simulink model "sampleModel1641_2_sub"  (R2023a)
settings: Solver=VariableStepAuto  StartTime=0.0  StopTime=10.0  RelTol=1e-3
libraries: hdlsllib x4, simulink x1
settings Model: Creator=user1  LastModifiedBy=user1

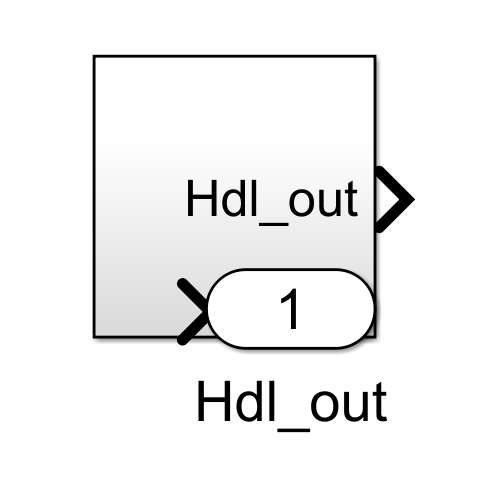
[thumbnail: Simulink's stored preview of the top-level diagram]
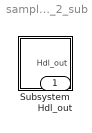
== system sampleModel1641_2_sub ==
  Subsystem : Subsystem
  Hdl_out : Outport  OutDataTypeStr=uint8

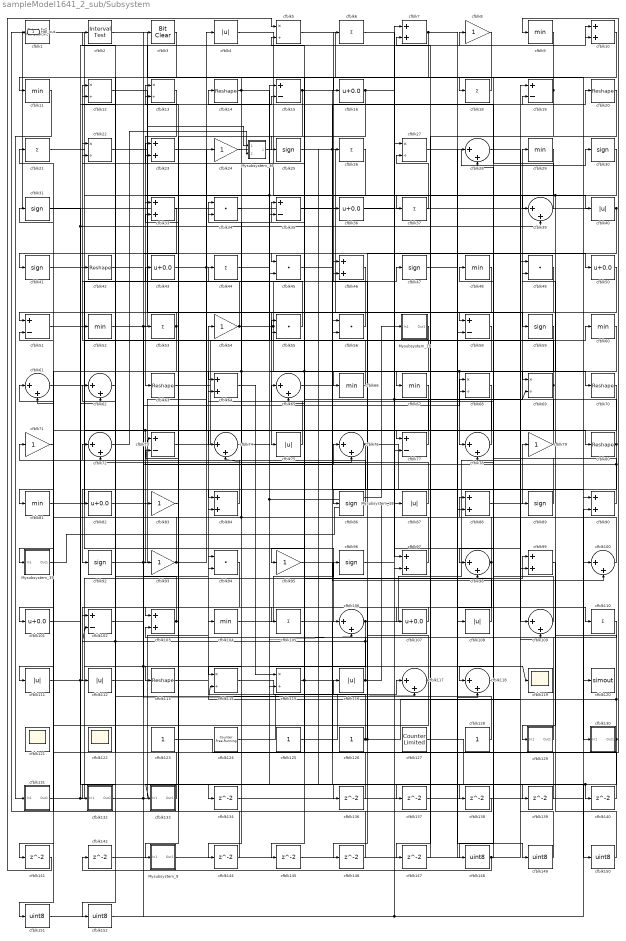
== system sampleModel1641_2_sub/Subsystem ==
  Mysubsystem_18 : Subsystem  TreatAsAtomicUnit=on  RTWFcnName=Mysubsystem_18
      settings: RTWFcnNameOpts=User specified  RTWFileNameOpts=Use function name
  Mysubsystem_19 : Subsystem  TreatAsAtomicUnit=on  RTWFcnName=Mysubsystem_19
      settings: RTWFcnNameOpts=User specified  RTWFileNameOpts=Use function name
  Mysubsystem_35 : Subsystem  TreatAsAtomicUnit=on  RTWFcnName=Mysubsystem_35
      settings: RTWFcnNameOpts=User specified  RTWFileNameOpts=Use function name
  Mysubsystem_36 : Subsystem  TreatAsAtomicUnit=on  RTWFcnName=Mysubsystem_36
      settings: RTWFcnNameOpts=User specified  RTWFileNameOpts=Use function name
  Mysubsystem_9 : Subsystem  TreatAsAtomicUnit=on  RTWFcnName=Mysubsystem_9
      settings: RTWFcnNameOpts=User specified  RTWFileNameOpts=Use function name
  cfblk1 : hdlsllib/Logic and Bit Operations/Detect Fall Nonpositive  vinit=0  OutDataTypeStr=uint8
  cfblk{7,10,23,33,46,64,84,88,90,97,99,103} (12 alike) : Sum  OutDataTypeStr=uint8
  cfblk{28,39,61..62,65,72,74,76,78,98,100,106,109,117..118} (15 alike) : Sum  Inputs=|++  OutDataTypeStr=uint8
  cfblk{16,36,43,50,82,101,107} (7 alike) : Bias  Bias=0.0  SaturateOnIntegerOverflow=off
  cfblk{15,19,35,51,58,73,77,102} (8 alike) : Sum  Inputs=+-  OutDataTypeStr=uint8
  cfblk{9,11,29,48,52,60,66..67,81,104} (10 alike) : MinMax  OutDataTypeStr=uint8
  cfblk{6,18,21,26,37,44,53,105,110} (9 alike) : Sum  Inputs=+  OutDataTypeStr=uint8
  cfblk{4,40,75,87,108,111..112,116} (8 alike) : Abs  OutDataTypeStr=uint8  SaturateOnIntegerOverflow=off
  cfblk{14,20,42,63,70,80,113} (7 alike) : Reshape
  cfblk{5,12..13,22,27,68..69,114..115} (9 alike) : Product  Inputs=*/  OutDataTypeStr=uint8  RndMeth=Zero  SaturateOnIntegerOverflow=on
  cfblk119 : Scope
  cfblk120 : ToWorkspace  VariableName=simout  SaveFormat=Timeseries  SampleTime=-1
  cfblk121 : Scope
      settings: Floating=on
  cfblk122 : Scope
      settings: Floating=on
  cfblk{123,125..126,128} (4 alike) : Constant  OutDataTypeStr=uint8  SampleTime=-1
  cfblk124 : hdlsllib/Sources/Counter Free-Running  NumBits=16  tsamp=-1
  cfblk127 : hdlsllib/Sources/Counter Limited  uplimit=7  tsamp=-1
  cfblk129 : Subsystem
      settings: LibrarySourceBlock=|
      | hdlsllib/Ports &
      | Subsystems/Subsystem
  cfblk130 : Subsystem
      settings: LibrarySourceBlock=|
      | hdlsllib/Ports &
      | Subsystems/Subsystem
  cfblk131 : Subsystem
      settings: LibrarySourceBlock=|
      | hdlsllib/Ports &
      | Subsystems/Subsystem
  cfblk132 : Subsystem
      settings: LibrarySourceBlock=|
      | hdlsllib/Ports &
      | Subsystems/Subsystem
  cfblk133 : Subsystem
      settings: LibrarySourceBlock=|
      | hdlsllib/Ports &
      | Subsystems/Subsystem
  cfblk{134,136..142,144..147} (12 alike) : Delay  SampleTime=1
  cfblk{148..152} (5 alike) : DataTypeConversion  OutDataTypeStr=uint8  SaturateOnIntegerOverflow=off  RndMeth=Floor
  cfblk2 : hdlsllib/Logic and Bit Operations/Interval Test  IntervalClosedRight=on  uplimit=0.5  IntervalClosedLeft=on  lowlimit=-0.5  OutDataTypeStr=uint8
  cfblk{8,24,54,71,79,83,93,95} (8 alike) : Gain  OutDataTypeStr=uint8
  cfblk{25,30..31,41,47,59,86,89,92,96} (10 alike) : Signum
  cfblk3 : simulink/Logic and Bit Operations/Bit Clear  iBit=0
      settings: LibrarySourceBlock=|
      | hdlsllib/Logic and Bit
      | Operations/Bit Clear
  cfblk{34,45,49,55..56,94} (6 alike) : DotProduct  OutDataTypeStr=uint8
  Hdl_out : Outport  OutDataTypeStr=uint8
  wires:
  cfblk126/1 -> cfblk54/1, cfblk46/2, cfblk89/1
  cfblk53/1 -> cfblk111/1, cfblk51/1
  cfblk64/1 -> cfblk115/1
  cfblk11/1 -> cfblk131/1(In1)
  cfblk116/1 -> cfblk87/1, cfblk13/2, cfblk102/2, cfblk52/1
  cfblk107/1 -> cfblk103/1
  cfblk45/1 -> cfblk10/1
  cfblk113/1 -> cfblk94/1
  cfblk81/1 -> cfblk60/1
  cfblk123/1 -> cfblk9/1
  cfblk52/1 -> cfblk10/2, cfblk117/2, cfblk8/1
  cfblk80/1 -> cfblk22/2, cfblk92/1
  cfblk96/1 -> cfblk7/1
  cfblk132/1(Out1) -> cfblk55/2, cfblk104/1
  cfblk41/1 -> cfblk106/1
  cfblk4/1 -> cfblk37/1
  cfblk58/1 -> cfblk78/1, cfblk102/1, cfblk74/2
  cfblk97/1 -> cfblk31/1
  cfblk51/1 -> cfblk80/1
  cfblk88/1 -> cfblk79/1
  cfblk84/1 -> cfblk71/1
  cfblk30/1 -> cfblk69/1, Mysubsystem_9/1(In1)
  cfblk102/1 -> cfblk94/2
  cfblk27/1 -> cfblk30/1
  cfblk59/1 -> cfblk145/1, cfblk101/1
  cfblk79/1 -> cfblk29/1
  cfblk36/1 -> cfblk39/1
  cfblk103/1 -> cfblk73/2, cfblk72/1
  cfblk1/1 -> cfblk90/1
  cfblk25/1 -> cfblk88/2, cfblk108/1
  cfblk46/1 -> cfblk75/1
  cfblk100/1 -> cfblk13/1, cfblk34/1
  cfblk12/1 -> cfblk58/1
  cfblk98/1 -> cfblk146/1, cfblk2/1
  cfblk108/1 -> cfblk35/1
  cfblk117/1 -> cfblk151/1, cfblk46/1
  cfblk19/1 -> cfblk77/1, cfblk16/1
  cfblk39/1 -> cfblk14/1
  cfblk9/1 -> cfblk58/2
  cfblk13/1 -> cfblk63/1
  cfblk76/1 -> cfblk84/1, cfblk100/1
  cfblk21/1 -> cfblk35/2
  cfblk130/1(Out1) -> cfblk84/2, cfblk114/2, cfblk140/1, cfblk133/1(In1)
  cfblk92/1 -> cfblk68/2, cfblk24/1
  cfblk131/1(Out1) -> cfblk6/1, cfblk99/1
  cfblk20/1 -> cfblk118/1
  cfblk16/1 -> cfblk105/1, cfblk97/1
  cfblk23/1 -> cfblk59/1
  cfblk111/1 -> cfblk113/1, cfblk15/2, cfblk39/2
  cfblk106/1 -> cfblk115/2, cfblk19/1
  cfblk73/1 -> cfblk15/1
  cfblk28/1 -> cfblk109/1
  cfblk7/1 -> cfblk110/1, cfblk25/1
  cfblk37/1 -> cfblk27/2
  cfblk112/1 -> cfblk76/1, cfblk119/1
  cfblk49/1 -> cfblk148/1
  cfblk93/1 -> cfblk21/1, cfblk47/1
  cfblk60/1 -> cfblk132/1(In1)
  cfblk55/1 -> cfblk12/1
  cfblk69/1 -> cfblk55/1, cfblk98/1
  cfblk2/1 -> cfblk18/1
  cfblk82/1 -> cfblk93/1
  cfblk18/1 -> cfblk11/1
  cfblk75/1 -> cfblk44/1
  cfblk29/1 -> cfblk107/1
  cfblk40/1 -> Hdl_out/1, cfblk86/1
  cfblk56/1 -> cfblk53/1
  cfblk50/1 -> cfblk82/1
  cfblk66/1 -> cfblk42/1
  cfblk10/1 -> cfblk78/2
  cfblk104/1 -> cfblk96/1
  cfblk99/1 -> cfblk129/1(In1)
  cfblk114/1 -> cfblk117/1
  cfblk48/1 -> cfblk66/1
  cfblk90/1 -> cfblk73/1, cfblk28/2
  cfblk129/1(Out1) -> cfblk23/1
  cfblk95/1 -> cfblk100/2
  cfblk65/1 -> cfblk56/2
  cfblk77/1 -> cfblk34/2
  cfblk86/1 -> cfblk61/1
  cfblk125/1 -> cfblk69/2, cfblk20/1
  cfblk94/1 -> cfblk112/1
  cfblk83/1 -> cfblk43/1
  cfblk89/1 -> cfblk68/1
  cfblk6/1 -> cfblk99/2
  cfblk67/1 -> cfblk95/1
  cfblk62/1 -> cfblk12/2
  cfblk61/1 -> cfblk4/1
  cfblk109/1 -> cfblk65/1
  cfblk118/1 -> cfblk88/1
  cfblk68/1 -> cfblk81/1, cfblk83/1
  cfblk3/1 -> cfblk152/1
  cfblk42/1 -> cfblk45/1
  cfblk43/1 -> cfblk77/2, cfblk50/1
  cfblk87/1 -> cfblk72/2
  cfblk15/1 -> cfblk70/1, cfblk33/1
  cfblk54/1 -> cfblk33/2, cfblk118/2, cfblk26/1
  cfblk124/1 -> cfblk116/1
  cfblk63/1 -> cfblk36/1
  cfblk128/1 -> cfblk62/1
  cfblk110/1 -> cfblk103/2
  cfblk115/1 -> cfblk5/2, cfblk19/2
  cfblk35/1 -> cfblk40/1
  cfblk8/1 -> cfblk74/1
  cfblk14/1 -> cfblk114/1, Mysubsystem_18/1(In1), cfblk106/2
  cfblk26/1 -> cfblk45/2, cfblk64/1
  cfblk33/1 -> cfblk41/1
  cfblk24/1 -> cfblk67/1
  cfblk78/1 -> cfblk64/2
  cfblk133/1(Out1) -> cfblk22/1
  cfblk101/1 -> cfblk62/2
  cfblk74/1 -> cfblk144/1, cfblk76/2
  cfblk5/1 -> cfblk130/1(In1)
  cfblk34/1 -> cfblk134/1
  cfblk134/1 -> cfblk90/2
  cfblk44/1 -> cfblk136/1
  cfblk136/1 -> cfblk56/1
  cfblk31/1 -> cfblk137/1
  cfblk137/1 -> cfblk28/1
  cfblk105/1 -> cfblk138/1
  cfblk138/1 -> cfblk1/1
  cfblk139/1 -> cfblk51/2
  cfblk140/1 -> cfblk65/2
  cfblk71/1 -> cfblk141/1
  cfblk141/1 -> cfblk5/1
  cfblk142/1 -> cfblk109/2
  cfblk144/1 -> cfblk23/2
  cfblk145/1 -> cfblk98/2
  cfblk146/1 -> cfblk61/2
  cfblk70/1 -> cfblk147/1
  cfblk147/1 -> cfblk7/2
  cfblk148/1 -> cfblk48/1, cfblk142/1
  cfblk47/1 -> cfblk149/1
  cfblk149/1 -> cfblk49/1
  cfblk127/1 -> cfblk150/1
  cfblk150/1 -> cfblk49/2
  cfblk151/1 -> cfblk3/1
  cfblk152/1 -> cfblk97/2, cfblk120/1
  Mysubsystem_9/1(Out1) -> cfblk27/1
  Mysubsystem_18/1(Out1) -> Mysubsystem_19/1(In1)
  Mysubsystem_19/1(Out1) -> Mysubsystem_35/1(In1)
  Mysubsystem_35/1(Out1) -> Mysubsystem_18/2(In2)
  cfblk22/1 -> Mysubsystem_36/1(In1)
  cfblk72/1 -> Mysubsystem_36/2(In2)
  Mysubsystem_36/1(Out1) -> cfblk139/1

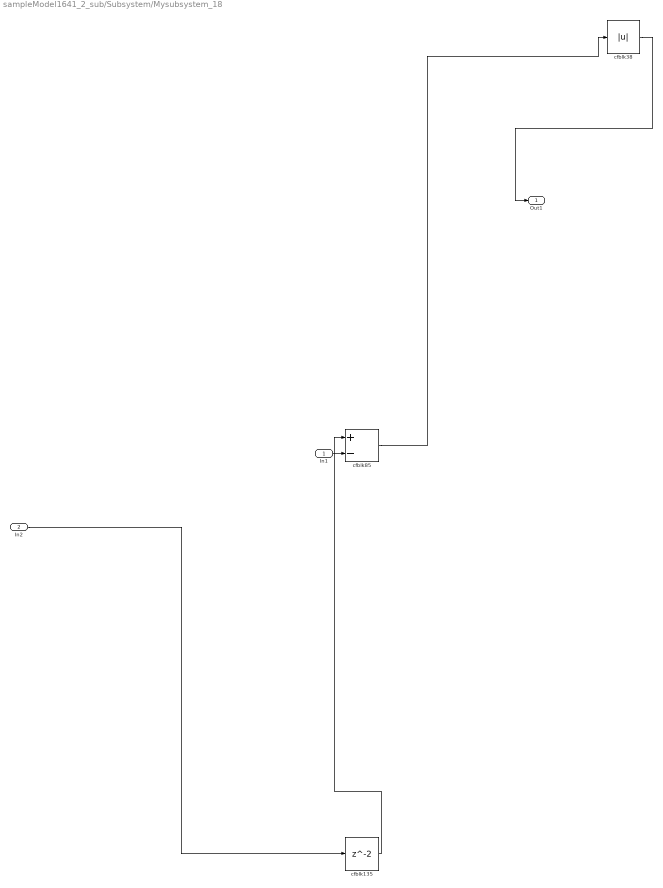
== system sampleModel1641_2_sub/Subsystem/Mysubsystem_18 ==
  In1 : Inport
  In2 : Inport  Port=2
  cfblk135 : Delay  SampleTime=1
  cfblk38 : Abs  SaturateOnIntegerOverflow=off
  cfblk85 : Sum  Inputs=+-
  Out1 : Outport
  wires:
  In1/1 -> cfblk85/2
  cfblk38/1 -> Out1/1
  cfblk85/1 -> cfblk38/1
  In2/1 -> cfblk135/1
  cfblk135/1 -> cfblk85/1

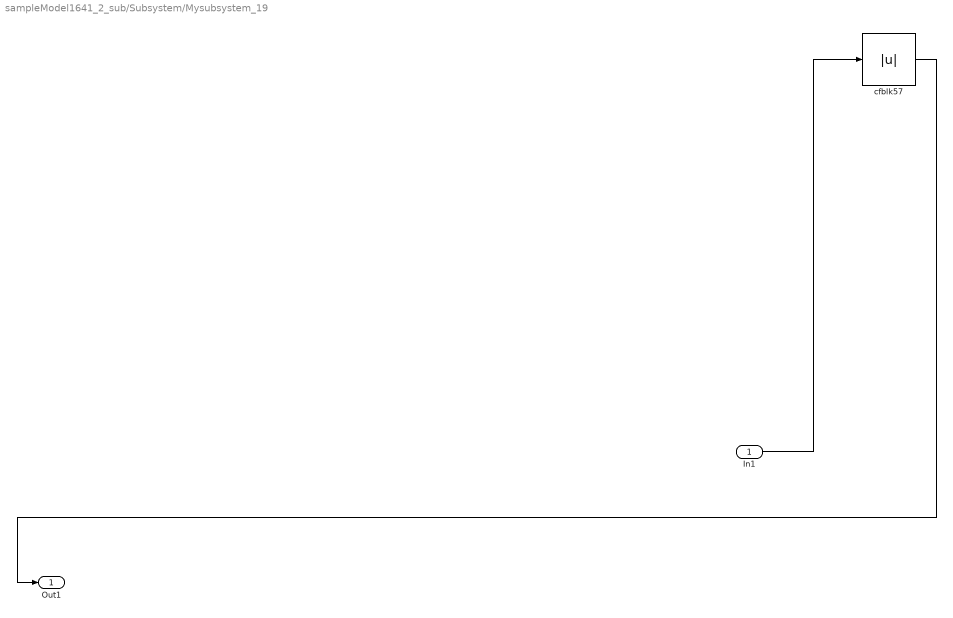
== system sampleModel1641_2_sub/Subsystem/Mysubsystem_19 ==
  In1 : Inport
  cfblk57 : Abs  SaturateOnIntegerOverflow=off
  Out1 : Outport
  wires:
  In1/1 -> cfblk57/1
  cfblk57/1 -> Out1/1

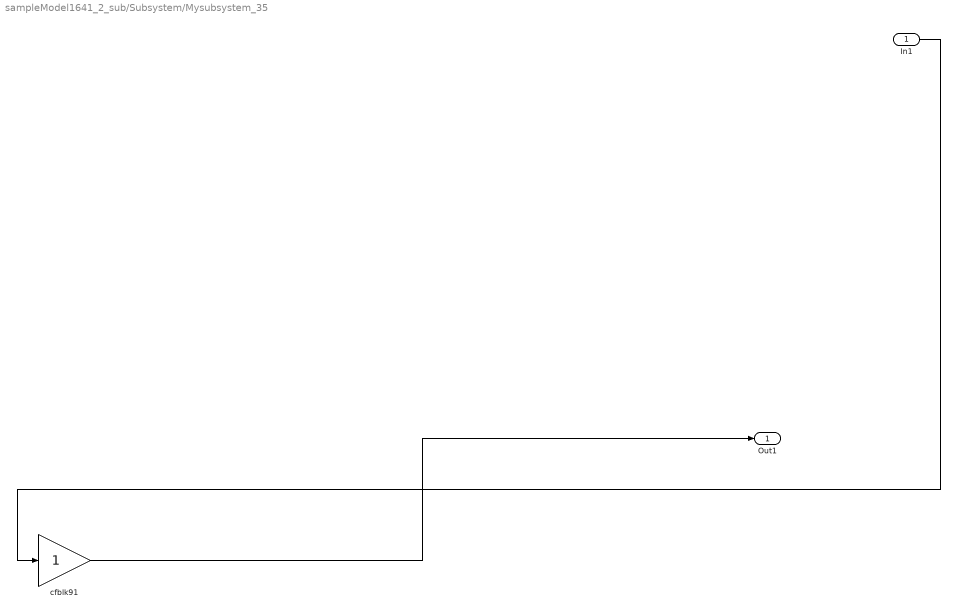
== system sampleModel1641_2_sub/Subsystem/Mysubsystem_35 ==
  In1 : Inport
  cfblk91 : Gain
  Out1 : Outport
  wires:
  In1/1 -> cfblk91/1
  cfblk91/1 -> Out1/1

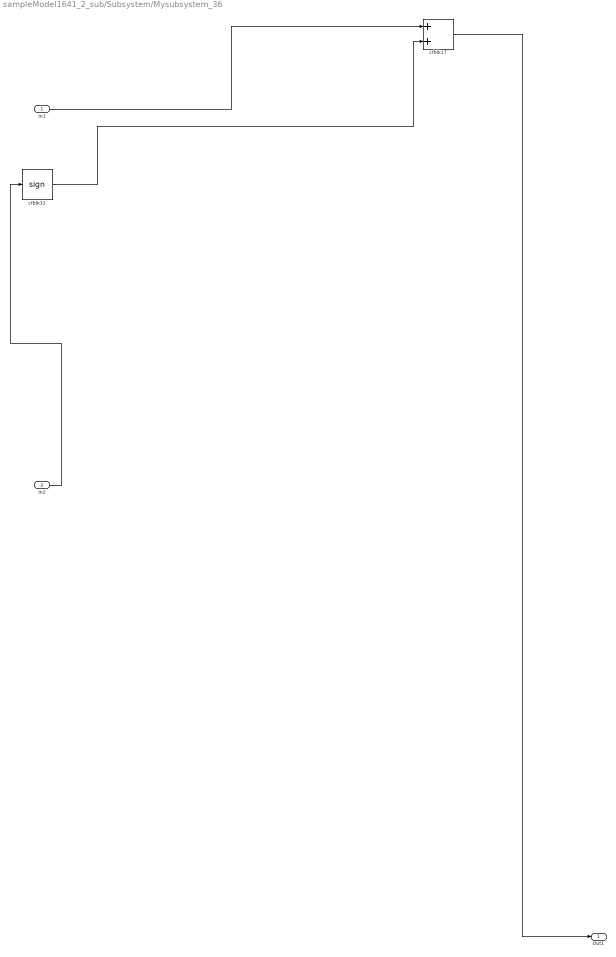
== system sampleModel1641_2_sub/Subsystem/Mysubsystem_36 ==
  In1 : Inport
  In2 : Inport  Port=2
  cfblk17 : Sum
  cfblk32 : Signum
  Out1 : Outport
  wires:
  cfblk17/1 -> Out1/1
  In1/1 -> cfblk17/1
  In2/1 -> cfblk32/1
  cfblk32/1 -> cfblk17/2

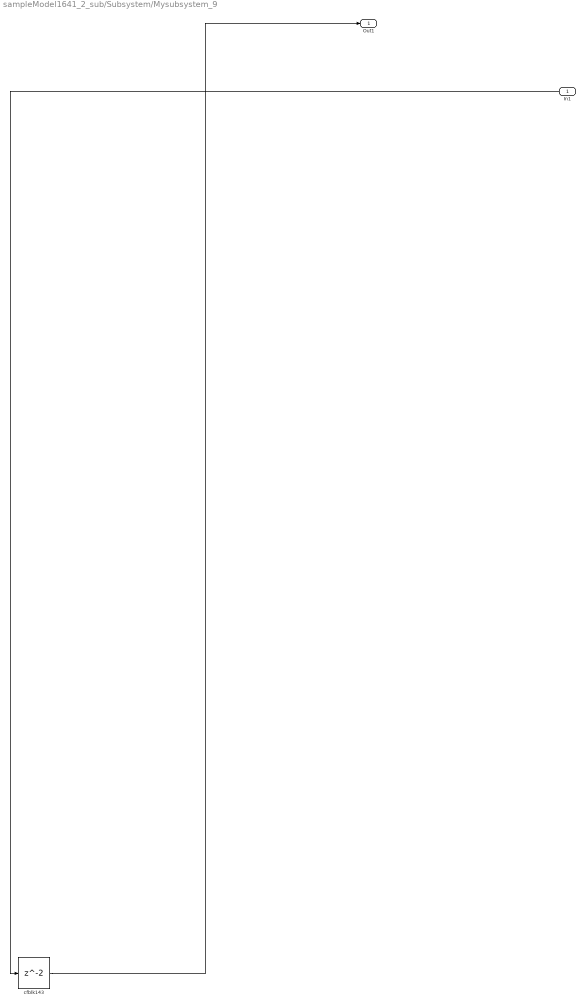
== system sampleModel1641_2_sub/Subsystem/Mysubsystem_9 ==
  In1 : Inport
  cfblk143 : Delay  SampleTime=1
  Out1 : Outport
  wires:
  cfblk143/1 -> Out1/1
  In1/1 -> cfblk143/1

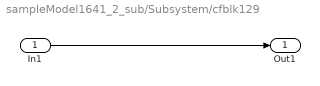
== system sampleModel1641_2_sub/Subsystem/cfblk129 ==
  In1 : Inport
  Out1 : Outport
  wires:
  In1/1 -> Out1/1

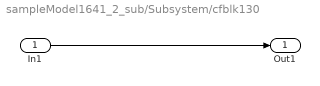
== system sampleModel1641_2_sub/Subsystem/cfblk130 ==
  In1 : Inport
  Out1 : Outport
  wires:
  In1/1 -> Out1/1

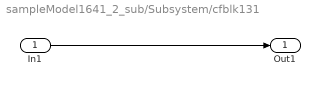
== system sampleModel1641_2_sub/Subsystem/cfblk131 ==
  In1 : Inport
  Out1 : Outport
  wires:
  In1/1 -> Out1/1

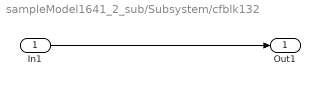
== system sampleModel1641_2_sub/Subsystem/cfblk132 ==
  In1 : Inport
  Out1 : Outport
  wires:
  In1/1 -> Out1/1

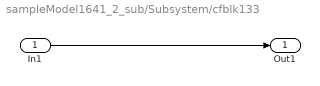
== system sampleModel1641_2_sub/Subsystem/cfblk133 ==
  In1 : Inport
  Out1 : Outport
  wires:
  In1/1 -> Out1/1
